simulink model "verify_Enthalpy2Temperature_mdl"  (R2018b)
settings: Solver=VariableStepDiscrete  StartTime=0.0  StopTime=10.0  MaxStep=0.1  RelTol=1e-3  EnableMultiTasking=on
libraries: carnot x3, simulink x1
settings Model: Creator=drhf  LastModifiedBy=drhf
settings DataIOCC: LimitDataPoints=on  SaveFormat=Array
settings OptimizationCC: ExpressionDepthLimit=2147483647  LifeSpan=inf
settings DebuggingCC: UnderspecifiedInitializationDetection=Classic  MergeDetectMultiDrivingBlocksExec=none  SolverPrmCheckMsg=warning  StateNameClashWarn=warning  SFUnexpectedBacktrackingDiag=warning  SFNoUnconditionalDefaultTransitionDiag=warning  SFExecutionAtInitializationDiag=none
settings HardwareCC: ProdBitPerPointer=32  ProdBitPerSizeT=32  ProdBitPerPtrDiffT=32  ProdLargestAtomicFloat=None  ProdIntDivRoundTo=Undefined  ProdEndianess=Unspecified  ProdWordSize=32  ProdHWDeviceType=32-bit Generic
settings ModelReferenceCC: PropagateSignalLabelsOutOfModel=off
settings SFSimCC: SimUseLocalCustomCode=off
settings RTWCC: RTWUseLocalCustomCode=off
settings CodeAppCC: StateflowObjectComments=on
settings GRTTargetCC: TargetLangStandard=C89/C90 (ANSI)  GeneratePreprocessorConditionals=Disable all  CombineOutputUpdateFcns=off  GRTInterface=on
settings ConfigComp: CovMetricSettings=dw  CovHtmlReporting=on  CovSaveCumulativeToWorkspaceVar=on  CovSaveSingleToWorkspaceVar=on  CovExternalEMLEnable=off

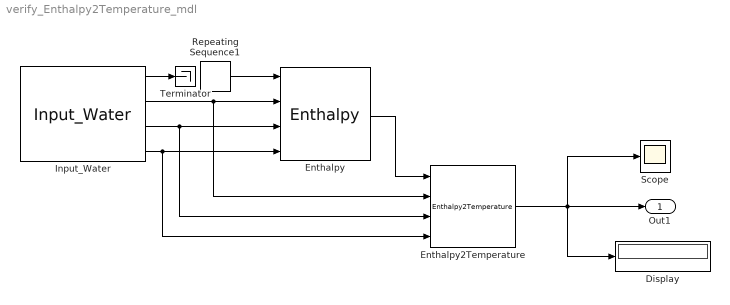
== system verify_Enthalpy2Temperature_mdl ==
  Display : Display
  Enthalpy : carnot/Basic/Material_Properties/Enthalpy  VariantControl=CarlibClassic  INPUTARGUMENTS=state variables (classic)  DEBUGLEVEL=WARNINGLEVEL  MAXTOTALMESSAGES=inf  MAXCONSECUTIVEMESSAGES=inf  WRITETOFILE=0  FILENAME='errors.txt'
  Enthalpy2Temperature : carnot/Basic/Material_Properties/Enthalpy2Temperature  VariantControl=CarlibClassic  DEBUGLEVEL=WARNINGLEVEL  MAXTOTALMESSAGES=inf  MAXCONSECUTIVEMESSAGES=inf  WRITETOFILE=0  FILENAME='errors.txt'
  Input_Water : carnot/Basic/Material_Properties/Input_Water  T=20  p=2e6  xd=0
  Repeating Sequence1 : simulink/Sources/Repeating Sequence  rep_seq_t=[0:10 11]  rep_seq_y=[0.01 5:5:50 50]
  Scope : Scope
  Terminator : Terminator
  Out1 : Outport
  wires:
  Enthalpy2Temperature/1 -> Scope/1, Display/1, Out1/1
  Input_Water/2 -> Enthalpy2Temperature/2, Enthalpy/2
  Input_Water/3 -> Enthalpy2Temperature/3, Enthalpy/3
  Input_Water/4 -> Enthalpy2Temperature/4, Enthalpy/4
  Input_Water/1 -> Terminator/1
  Enthalpy/1 -> Enthalpy2Temperature/1
  Repeating Sequence1/1 -> Enthalpy/1
